simulink model "manipulator2c12"  (Simulink 10.0)
settings: Solver=FixedStepAuto  StartTime=0.0  StopTime=10.2557  FixedStep=0.001  RelTol=1e-3
settings Model: Creator=dell  LastModifiedBy=JOHN WICK
settings DataIOCC: SaveFormat=Dataset
settings OptimizationCC: LifeSpan=auto
settings DebuggingCC: UnderspecifiedInitializationDetection=Simplified  MergeDetectMultiDrivingBlocksExec=error  SFUnexpectedBacktrackingDiag=error  SFNoUnconditionalDefaultTransitionDiag=error  SFExecutionAtInitializationDiag=warning
settings HardwareCC: ProdBitPerPointer=64  ProdBitPerSizeT=64  ProdBitPerPtrDiffT=64  ProdLargestAtomicFloat=Float  ProdIntDivRoundTo=Zero  ProdEndianess=LittleEndian  ProdWordSize=64  ProdHWDeviceType=Intel->x86-64 (Windows64)
settings ModelReferenceCC: PropagateSignalLabelsOutOfModel=on
settings GRTTargetCC: TargetLangStandard=C99 (ISO)  CombineOutputUpdateFcns=on  GRTInterface=off
settings ConfigComp: CovMetricSettings=dwe  CovHtmlReporting=off  CovSaveCumulativeToWorkspaceVar=off  CovSaveSingleToWorkspaceVar=off

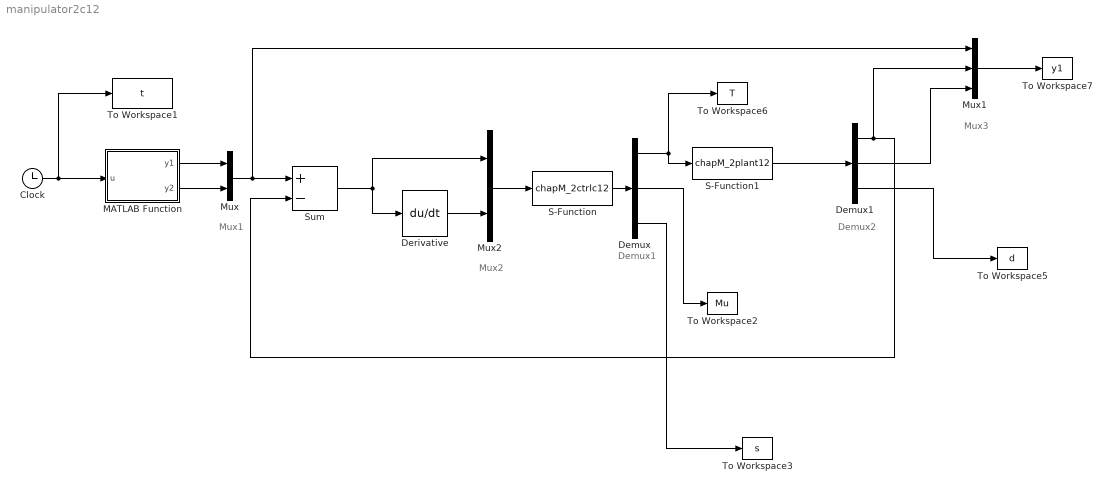
== system manipulator2c12 ==
  note: Demux2
  note: Mux3
  note: Demux1
  note: Mux2
  note: Mux1
  Clock : Clock
  Demux : Demux  Outputs=3
  Demux1 : Demux  Outputs=3
  Derivative : Derivative
  MATLAB Function : MATLAB Function  TreatAsAtomicUnit=on
  Mux : Mux  Inputs=2
  Mux1 : Mux  Inputs=3
  Mux2 : Mux  Inputs=2
  S-Function : S-Function  FunctionName=chapM_2ctrlc12  SFunctionDeploymentMode=off  EnableBusSupport=off
  S-Function1 : S-Function  FunctionName=chapM_2plant12  SFunctionDeploymentMode=off  EnableBusSupport=off
  Sum : Sum  Inputs=+-  SaturateOnIntegerOverflow=on  InputSameDT=on  OutDataTypeStr=Inherit: Same as first input
  To Workspace1 : ToWorkspace  VariableName=t  SampleTime=-1
  To Workspace2 : ToWorkspace  VariableName=Mu  SampleTime=-1
  To Workspace3 : ToWorkspace  VariableName=s  SampleTime=-1
  To Workspace5 : ToWorkspace  VariableName=d  SampleTime=-1
  To Workspace6 : ToWorkspace  VariableName=T  SampleTime=-1
  To Workspace7 : ToWorkspace  VariableName=y1  SampleTime=-1
  wires:
  MATLAB Function/2(y2) -> Mux/2
  MATLAB Function/1(y1) -> Mux/1
  S-Function/1 -> Demux/1
  Demux/1 -> S-Function1/1, To Workspace6/1
  S-Function1/1 -> Demux1/1
  Clock/1 -> To Workspace1/1, MATLAB Function/1(u)
  Mux2/1 -> S-Function/1
  Derivative/1 -> Mux2/2
  Mux1/1 -> To Workspace7/1
  Mux/1 -> Mux1/1, Sum/1
  Sum/1 -> Mux2/1, Derivative/1
  Demux/2 -> To Workspace2/1
  Demux1/3 -> To Workspace5/1
  Demux1/1 -> Mux1/2, Sum/2
  Demux1/2 -> Mux1/3
  Demux/3 -> To Workspace3/1

== matlab function MATLAB Function ==
  data: u input double; y1 output double; y2 output double
function [y1,y2]=fcn(u)
tnode=[0	2.380632392	3.505666959	4.275059855	6.612705584	7.88863381	10.25572392];

curve1=[-0.015247503	0.073099385	0	0	0
0.02429041	-0.303401555	1.344465498	-2.13378541	1.269939666
-0.012466572	0.21202939	-1.365928351	4.200706699	-4.281715256
0.000477439	-0.009316298	0.053470747	0.155362631	0.04180675
-0.003434695	0.094162857	-0.972945034	4.680286207	-7.438690099
0.011421834	-0.374628006	4.57423414	-24.49282391	50.09530561];

curve2=[-0.001880225	0.009296327	-6.76E-17	0	0.523598776
-0.001964466	0.010098519	-0.002864585	0.00454635	0.520892979
0.013579766	-0.20787309	1.143339217	-2.674259516	2.868643282
-0.003234178	0.079649387	-0.700424484	2.580540605	-2.747502979
-0.001028148	0.021298061	-0.121634275	0.028961104	1.470708026
0.00292008	-0.103286436	1.352567943	-7.723999868	16.76077554];

if u>=tnode(1)&&u<tnode(2)
    y1=curve1(1,:)*[u^4,u^3,u^2,u,1]';
    y2=curve2(1,:)*[u^4,u^3,u^2,u,1]';
elseif u>=tnode(2)&&u<tnode(3)
    y1=curve1(2,:)*[u^4,u^3,u^2,u,1]';
    y2=curve2(2,:)*[u^4,u^3,u^2,u,1]';
elseif u>=tnode(3)&&u<tnode(4)
    y1=curve1(3,:)*[u^4,u^3,u^2,u,1]';
    y2=curve2(3,:)*[u^4,u^3,u^2,u,1]';
elseif u>=tnode(4)&&u<tnode(5)
    y1=curve1(4,:)*[u^4,u^3,u^2,u,1]';
    y2=curve2(4,:)*[u^4,u^3,u^2,u,1]';
elseif u>=tnode(5)&&u<tnode(6)
    y1=curve1(5,:)*[u^4,u^3,u^2,u,1]';
    y2=curve2(5,:)*[u^4,u^3,u^2,u,1]';
else u>=tnode(6)&&u<=tnode(7)
    y1=curve1(6,:)*[u^4,u^3,u^2,u,1]';
    y2=curve2(6,:)*[u^4,u^3,u^2,u,1]';
end
